simulink model "produzione_regolato"  (Simulink 7.7)
settings: Solver=FixedStepDiscrete  StartTime=0.0  StopTime=10.0  RelTol=1e-9  AbsTol=1e-9
values from neighbouring files (symbols this model uses):
  A = [0 1; 0 -h/J]    [antenna.m]    (also in produzione.m = [0 (1-alpha)*(1-beta2); 1-beta1 0]; serbatoi.m = [-d1 0; d1 -d2])
  Atilde = [-h/J 0; -1 0]    [motore.m]    (also in produzione.m = [0 (1-alpha)*(1-beta2) 0; 1-beta1 0 0; 0 -alpha*(1-beta2) 1])
  b = [0; 1/J]    [antenna.m]    (also in produzione.m = [1; 0]; serbatoi.m = [1; 0])
  btilde = [nu/J; 0]    [motore.m]    (also in produzione.m = [1; 0; 0])
  c = [1 0]    [antenna.m]    (also in produzione.m = [0 alpha*(1-beta2)]; serbatoi.m = [0 d2])
  ctilde = [0 1]    [motore.m]    (also in produzione.m = [0 0 1])
  d = 0    [antenna.m]    (also in produzione.m; serbatoi.m)
  dist = -3    [motore.m]    (also in produzione.m = 3)
  k = [k1 k2]    [antenna.m]    (also in motore.m; produzione.m = [k1 k2 k3]; serbatoi.m)
  l = [l1; l2]    [antenna.m]    (also in motore.m; produzione.m = [l1; l2; l3]; serbatoi.m)
  x0 = [-0.5 0]'    [antenna.m]    (also in produzione.m = [1 0]'; serbatoi.m = [1 0]')
  xcap0 = [0 0]'    [antenna.m]    (also in produzione.m; serbatoi.m)
  y0 = 0.5    [antenna.m]    (also in motore.m = 5; produzione.m = 50; serbatoi.m = 5)
undefined symbols (not defined in the file or in its folder): DiscIntNeverNeededParam
settings Model: Creator=fabio  LastModifiedBy=fabio

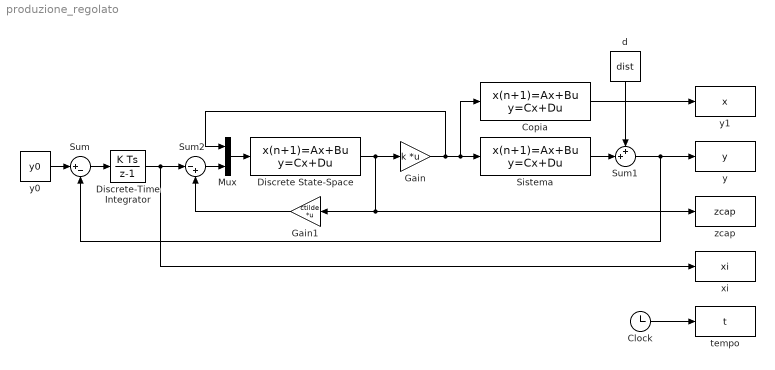
== system produzione_regolato ==
  Clock : Clock
  Copia : DiscreteStateSpace  A=A  B=b  C=[1 0; 0 1]  D=[0; 0]  X0=x0
  Discrete State-Space : DiscreteStateSpace  A=Atilde  B=[btilde l]  C=eye(3)  D=[0 0; 0 0; 0 0]  X0=[xcap0; 0]
  Discrete-Time Integrator : DiscreteIntegrator  ICPrevOutput=DiscIntNeverNeededParam  ICPrevScaledInput=DiscIntNeverNeededParam
  Gain : Gain  Gain=k  Multiplication=Matrix(K*u)
  Gain1 : Gain  Gain=ctilde  Multiplication=Matrix(K*u)
  Mux : Mux  Inputs=2
  Sistema : DiscreteStateSpace  A=A  B=b  C=c  D=d  X0=x0
  Sum : Sum  Inputs=|+-
  Sum1 : Sum  Inputs=++|
  Sum2 : Sum  Inputs=|-+
  d : Constant  Value=dist
  tempo : ToWorkspace  VariableName=t  SampleTime=-1  SaveFormat=Array
  xi : ToWorkspace  VariableName=xi  SampleTime=-1  SaveFormat=Array
  y : ToWorkspace  VariableName=y  SampleTime=-1  SaveFormat=Array
  y0 : Constant  Value=y0
  y1 : ToWorkspace  VariableName=x  SampleTime=-1  SaveFormat=Array
  zcap : ToWorkspace  VariableName=zcap  SampleTime=-1  SaveFormat=Array
  wires:
  y0/1 -> Sum/1
  Sum/1 -> Discrete-Time Integrator/1
  Discrete State-Space/1 -> zcap/1, Gain1/1, Gain/1
  Mux/1 -> Discrete State-Space/1
  Clock/1 -> tempo/1
  Gain1/1 -> Sum2/2
  Discrete-Time Integrator/1 -> Sum2/1, xi/1
  Sum2/1 -> Mux/2
  Sum1/1 -> y/1, Sum/2
  d/1 -> Sum1/1
  Sistema/1 -> Sum1/2
  Gain/1 -> Mux/1, Sistema/1, Copia/1
  Copia/1 -> y1/1
